simulink model "sfbk_ip_EV3"  (R2014b)
settings: Solver=FixedStepDiscrete  SolverMode=SingleTasking  StartTime=0.0  StopTime=60  FixedStep=h  RelTol=1e-3
values from neighbouring files (symbols this model uses):
  h = t(2) - t(1)    [ident_pend.m]    (also in rotary_ip_lq.m = 0.01)
  K = 0.00012892    [RotatedPendulumParams.m]    (also in rotary_ip_lq.m = - lqr(A,B,Q,R))
  Tf1 = 0.06    [rotary_ip_lq.m]
  Tf2 = 0.025    [ident_pend.m]    (also in rotary_ip_lq.m = 0.06)
libraries: legoev3lib x4
PreSaveFcn:
  | set_param(gcs, 'location', [15 50 815 560])
settings Model: FPTRunName=Active  SimulationMode=external  ExtModeTrigDuration=2  Creator=The MathWorks Inc.  LastModifiedBy=kawata
settings DataIOCC: SignalLoggingSaveFormat=ModelDataLogs
settings OptimizationCC: ExpressionDepthLimit=2147483647  OptimizeModelRefInitCode=on  LifeSpan=Inf
settings DebuggingCC: UnderspecifiedInitializationDetection=Classic  MergeDetectMultiDrivingBlocksExec=none  SolverPrmCheckMsg=none  InheritedTsInSrcMsg=none  FcnCallInpInsideContextMsg=EnableAllAsWarning  StateNameClashWarn=warning
settings HardwareCC: ProdLargestAtomicInteger=Long  ProdLargestAtomicFloat=Float  ProdEndianess=LittleEndian  ProdHWDeviceType=ARM Compatible->ARM 9
settings RTWCC: SystemTargetFile=realtime.tlc  GenerateMakefile=off  TemplateMakefile=realtime.tmf  Description=Real-Time Toolbox  RTWVerbose=off  ProcessScript=realtime_make_rtw_hook
settings CodeAppCC: CustomSymbolStrType=$N$R$M  InternalIdentifier=Classic
settings STFCustomTargetCC: TargetLibSuffix=.a  GenerateSampleERTMain=on  ERTCustomFileBanners=on  SupportNonInlinedSFcns=off  SupportVariableSizeSignals=on  MATLABClassNameForMDSCustomization=Simulink.SoftwareTarget.ERTCustomization  GRTInterface=off  SystemTargetFile=realtime.tlc
settings ERTTargetCC: GenerateSampleERTMain=on  ParMdlRefBuildCompliant=off  CompOptLevelCompliant=off  ConcurrentExecutionCompliant=off  CombineOutputUpdateFcns=off  ERTFirstTimeCompliant=off  SupportContinuousTime=on  SupportVariableSizeSignals=on  ModelStepFunctionPrototypeControlCompliant=off  CPPClassGenCompliant=off  ExtMode=on  ExtModeMexArgs=0 12 9600  InlinedParameterPlacement=NonHierarchical  ERTSrcFileBannerTemplate=realtime_code_template.cgt  ERTHdrFileBannerTemplate=realtime_code_template.cgt  ERTDataSrcFileTemplate=realtime_code_template.cgt  ERTDataHdrFileTemplate=realtime_code_template.cgt  ERTCustomFileTemplate=realtime_file_process.tlc

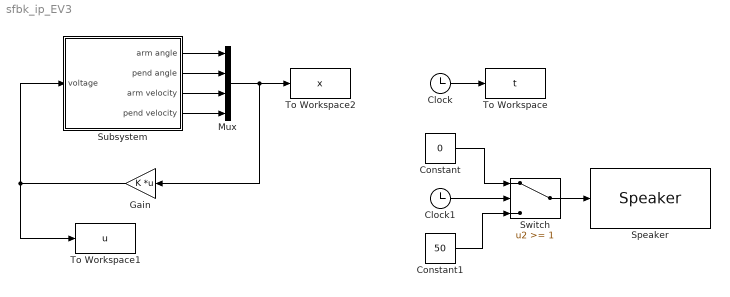
== system sfbk_ip_EV3 ==
  Clock : Clock
  Clock1 : Clock
  Constant : Constant  Value=0
  Constant1 : Constant  Value=50
  Gain : Gain  Gain=K  Multiplication=Matrix(K*u)
  Mux : Mux
  Speaker : legoev3lib/Speaker  sinputMode=Volume only  sspeakerFreq=100  sspeakerVolume=50  sspeakerDuration=1000
  Subsystem : Subsystem
  Switch : Switch  Threshold=1
  To Workspace : ToWorkspace  VariableName=t  SampleTime=-1
  To Workspace1 : ToWorkspace  VariableName=u  SampleTime=-1
  To Workspace2 : ToWorkspace  VariableName=x  SampleTime=-1
  wires:
  Subsystem/1(arm angle) -> Mux/1
  Subsystem/2(pend angle) -> Mux/2
  Subsystem/3(arm velocity) -> Mux/3
  Subsystem/4(pend velocity) -> Mux/4
  Clock/1 -> To Workspace/1
  Clock1/1 -> Switch/2
  Switch/1 -> Speaker/1
  Mux/1 -> Gain/1, To Workspace2/1
  Gain/1 -> Subsystem/1(voltage), To Workspace1/1
  Constant/1 -> Switch/1
  Constant1/1 -> Switch/3

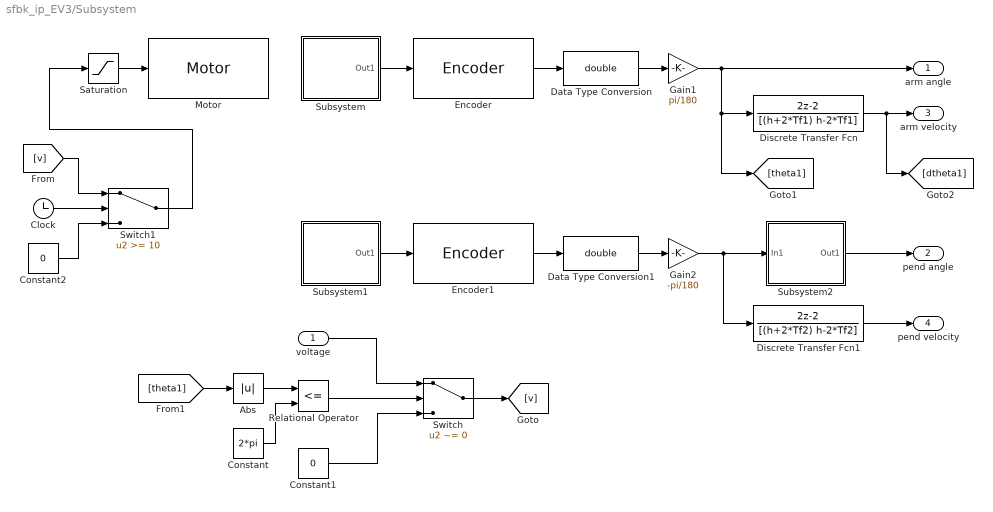
== system sfbk_ip_EV3/Subsystem ==
  voltage : Inport
  Abs : Abs  SaturateOnIntegerOverflow=on
  Clock : Clock
  Constant : Constant  Value=2*pi
  Constant1 : Constant  Value=0
  Constant2 : Constant  Value=0
  Data Type Conversion : DataTypeConversion  OutDataTypeStr=double  RndMeth=Simplest
  Data Type Conversion1 : DataTypeConversion  OutDataTypeStr=double  RndMeth=Simplest
  Discrete Transfer Fcn : DiscreteTransferFcn  Numerator=[2 -2]  Denominator=[(h+2*Tf1) h-2*Tf1]  SampleTime=h
  Discrete Transfer Fcn1 : DiscreteTransferFcn  Numerator=[2 -2]  Denominator=[(h+2*Tf2) h-2*Tf2]  SampleTime=h
  Encoder : legoev3lib/Encoder  portNumber=A  opMode=Reset by external signal  sampleTime=h
  Encoder1 : legoev3lib/Encoder  portNumber=C  opMode=Reset by external signal  sampleTime=h
  Gain1 : Gain  Gain=pi/180
  Gain2 : Gain  Gain=-pi/180
  Motor : legoev3lib/Motor  sportNumber=A  sstopAction=Brake
  Relational Operator : RelationalOperator  Operator=<=  InputSameDT=on
  Saturation : Saturate  UpperLimit=100  LowerLimit=-100
  Subsystem : Subsystem
  Subsystem1 : Subsystem
  Subsystem2 : Subsystem
  Switch : Switch  Criteria=u2 ~= 0
  Switch1 : Switch  Threshold=10
  arm angle : Outport
  pend angle : Outport  Port=2
  arm velocity : Outport  Port=3
  pend velocity : Outport  Port=4
  wires:
  Encoder1/1 -> Data Type Conversion1/1
  Encoder/1 -> Data Type Conversion/1
  Discrete Transfer Fcn/1 -> [dtheta1], arm velocity/1
  Data Type Conversion/1 -> Gain1/1
  Data Type Conversion1/1 -> Gain2/1
  Saturation/1 -> Motor/1
  Gain1/1 -> arm angle/1, [theta1], Discrete Transfer Fcn/1
  Relational Operator/1 -> Switch/2
  Abs/1 -> Relational Operator/1
  Constant/1 -> Relational Operator/2
  Switch/1 -> [v]
  [theta1] -> Abs/1
  Gain2/1 -> Discrete Transfer Fcn1/1, Subsystem2/1(In1)
  Discrete Transfer Fcn1/1 -> pend velocity/1
  Constant1/1 -> Switch/3
  voltage/1 -> Switch/1
  Switch1/1 -> Saturation/1
  [v] -> Switch1/1
  Clock/1 -> Switch1/2
  Constant2/1 -> Switch1/3
  Subsystem2/1(Out1) -> pend angle/1
  Subsystem1/1(Out1) -> Encoder1/1
  Subsystem/1(Out1) -> Encoder/1

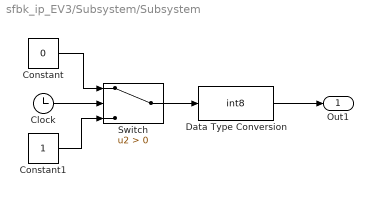
== system sfbk_ip_EV3/Subsystem/Subsystem ==
  Clock : Clock
  Constant : Constant  Value=0
  Constant1 : Constant
  Data Type Conversion : DataTypeConversion  OutDataTypeStr=int8  RndMeth=Simplest
  Switch : Switch  Criteria=u2 > Threshold
  Out1 : Outport
  wires:
  Data Type Conversion/1 -> Out1/1
  Constant1/1 -> Switch/3
  Constant/1 -> Switch/1
  Switch/1 -> Data Type Conversion/1
  Clock/1 -> Switch/2

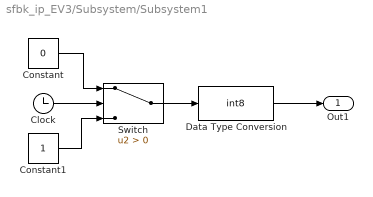
== system sfbk_ip_EV3/Subsystem/Subsystem1 ==
  Clock : Clock
  Constant : Constant  Value=0
  Constant1 : Constant
  Data Type Conversion : DataTypeConversion  OutDataTypeStr=int8  RndMeth=Simplest
  Switch : Switch  Criteria=u2 > Threshold
  Out1 : Outport
  wires:
  Clock/1 -> Switch/2
  Switch/1 -> Data Type Conversion/1
  Constant/1 -> Switch/1
  Constant1/1 -> Switch/3
  Data Type Conversion/1 -> Out1/1

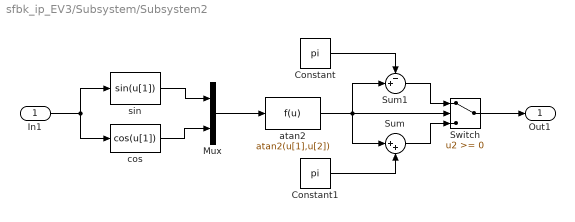
== system sfbk_ip_EV3/Subsystem/Subsystem2 ==
  In1 : Inport
  Constant : Constant  Value=pi
  Constant1 : Constant  Value=pi
  Mux : Mux  Inputs=2
  Sum : Sum  Inputs=|++  SaturateOnIntegerOverflow=on  InputSameDT=on  OutDataTypeStr=Inherit: Same as first input
  Sum1 : Sum  Inputs=-+|  SaturateOnIntegerOverflow=on  InputSameDT=on  OutDataTypeStr=Inherit: Same as first input
  Switch : Switch  SaturateOnIntegerOverflow=on  InputSameDT=on
  atan2 : Fcn  Expr=atan2(u[1],u[2])
  cos : Fcn  Expr=cos(u[1])
  sin : Fcn
  Out1 : Outport
  wires:
  Switch/1 -> Out1/1
  Constant/1 -> Sum1/1
  Sum/1 -> Switch/3
  Constant1/1 -> Sum/2
  Sum1/1 -> Switch/1
  atan2/1 -> Sum/1, Sum1/2, Switch/2
  In1/1 -> cos/1, sin/1
  sin/1 -> Mux/1
  cos/1 -> Mux/2
  Mux/1 -> atan2/1
